simulink model "closedloop_pid"  (Simulink 8.3)
settings: Solver=ode45  StartTime=0.0  StopTime=60  RelTol=1e-3
libraries: cstblocks x2, simulink x1
settings Model: Creator=henrik  LastModifiedBy=hg35a
settings DataIOCC: SignalLoggingName=sigsOut
settings OptimizationCC: ExpressionDepthLimit=2147483647  InitFltsAndDblsToZero=on
settings DebuggingCC: SaveWithParameterizedLinksMsg=none  SignalResolutionControl=TryResolveAllWithWarning  SolverPrmCheckMsg=none  MultiTaskDSMMsg=warning  MultiTaskCondExecSysMsg=none  FcnCallInpInsideContextMsg=UseLocalSettings
settings HardwareCC: TargetUnknown=on
settings RTWCC: IncludeERTFirstTime=on
settings GRTTargetCC: TargetFcnLib=ansi_tfl_tmw.mat  ModelReferenceCompliant=off  MatFileLogging=off

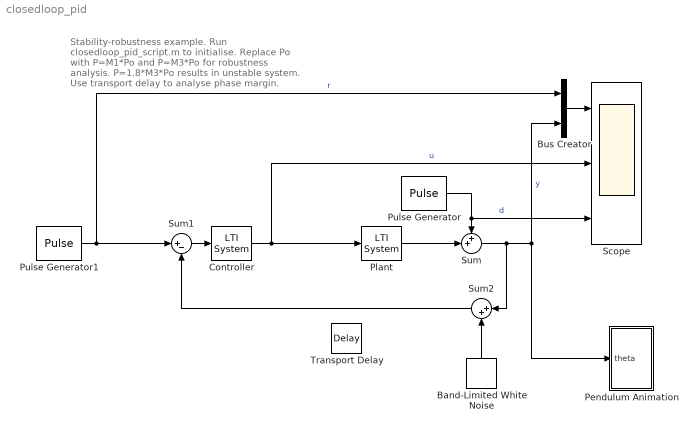
== system closedloop_pid ==
  note: Stability-robustness example.
      | Run closedloop_pid_script.m to initialise.
      | Replace Po with P=M1*Po and P=M3*Po
      | for robustness analysis.
      | P=1.8*M3*Po results in unstable system.
      | Use transport delay to analyse phase margin.
  Band-Limited White Noise : simulink/Sources/Band-Limited White Noise  Cov=[0.000001]*0  Ts=0.01  seed=[23341]
  Bus Creator : BusCreator  Inputs=2
  Controller : cstblocks/LTI System  sys=C  IC=[]
  Pendulum Animation : Subsystem
  Plant : cstblocks/LTI System  sys=Po  IC=[]
  Pulse Generator : DiscretePulseGenerator  PulseType=Time based  Amplitude=0.5  Period=60  PulseWidth=50  PhaseDelay=30
  Pulse Generator1 : DiscretePulseGenerator  PulseType=Time based  Amplitude=0.3  Period=10  PulseWidth=50
  Scope : Scope  NumInputPorts=3
      settings: YMin=0~-250~-1  YMax=0.3~50~1
  Sum : Sum  Inputs=++|  SaturateOnIntegerOverflow=on
  Sum1 : Sum  Inputs=|+-  SaturateOnIntegerOverflow=on
  Sum2 : Sum  Inputs=|++  SaturateOnIntegerOverflow=on
  Transport Delay : TransportDelay  DelayTime=0.03
  wires:
  Controller/1 -> Scope/2, Plant/1  "u"
  Pulse Generator/1 -> Sum/1, Scope/3  "d"
  Pulse Generator1/1 -> Bus Creator/1, Sum1/1  "r"
  Bus Creator/1 -> Scope/1
  Sum/1 -> Pendulum Animation/1(theta), Bus Creator/2, Sum2/1  "y"
  Sum1/1 -> Controller/1
  Sum2/1 -> Sum1/2
  Band-Limited White Noise/1 -> Sum2/2
  Plant/1 -> Sum/2

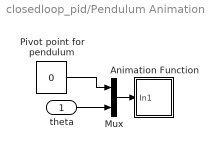
== system closedloop_pid/Pendulum Animation ==
  theta : Inport
  Animation Function : Subsystem  mask(Animation Block){ts=0.01}
      mask prompts: ts "Sample time:"
      mask Display: plot([.1,.9],[.9,.9],[.5,.2],[.9,.25],[.475,.475,.525,.525,.475],[.875,.925,.925,.875,.875])
  Mux : Mux  Inputs=2
  Pivot point for pendulum : Constant  Value=0
  wires:
  Mux/1 -> Animation Function/1(In1)
  Pivot point for pendulum/1 -> Mux/1
  theta/1 -> Mux/2

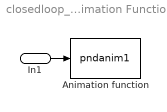
== system closedloop_pid/Pendulum Animation/Animation Function ==
  In1 : Inport
  Animation function : S-Function  FunctionName=pndanim1  Parameters=ts  EnableBusSupport=off
      settings: DeleteFcn=if ~isempty(findobj('type','figure','name','simppend Animation'));close('simppend Animation'); end;
  wires:
  In1/1 -> Animation function/1
